simulink model "RobotSimulation"  (R2018b)
settings: Solver=VariableStepAuto  StartTime=0.0  StopTime=1  RelTol=1e-3
values from neighbouring files (symbols this model uses):
  jointAngle = inverseKinematic.ComputeInverseKinematic(jointAngle, endPose)    [CartesianTrajectoryGeneration.m]
  jointAngleStart = [175.0; 145.0; 178.0; 90.0; 180.0; 215.0; 260.0]    [CartesianTrajectoryGeneration.m]
settings Model: Creator=olavoie  LastModifiedBy=olavoie

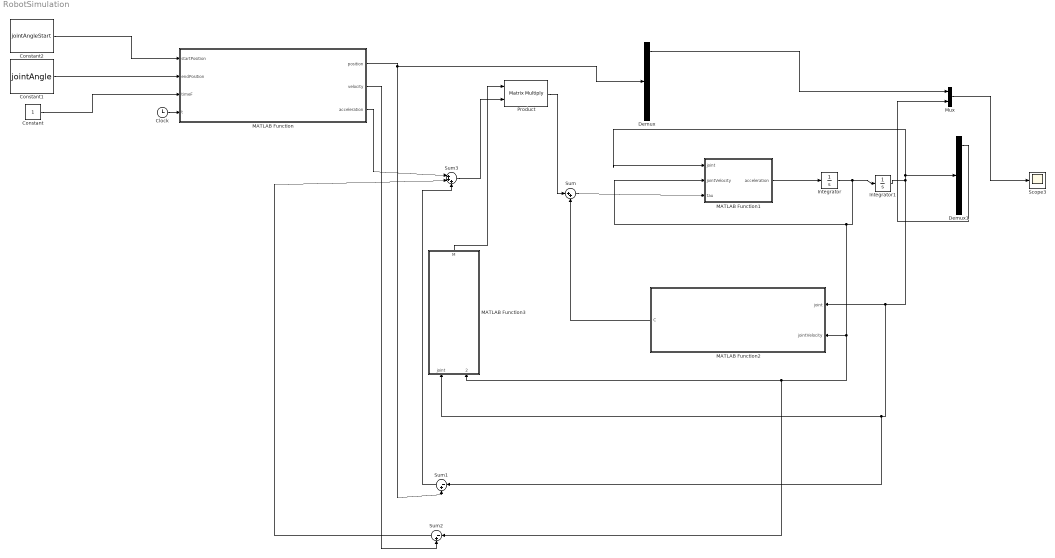
== system RobotSimulation ==
  Clock : Clock
  Constant : Constant
  Constant1 : Constant  Value=jointAngle
  Constant2 : Constant  Value=jointAngleStart
  Demux : Demux  Outputs=7
  Demux1 : Demux  Outputs=7
  Integrator : Integrator
  Integrator1 : Integrator  InitialCondition=175
  MATLAB Function : MATLAB Function  TreatAsAtomicUnit=on
  MATLAB Function1 : MATLAB Function  TreatAsAtomicUnit=on
  MATLAB Function2 : MATLAB Function  TreatAsAtomicUnit=on
  MATLAB Function3 : MATLAB Function  TreatAsAtomicUnit=on
  Mux : Mux  Inputs=2
  Product : Product  Multiplication=Matrix(*)
  Scope3 : Scope
  Sum : Sum  Inputs=|++
  Sum1 : Sum  Inputs=|-+
  Sum2 : Sum  Inputs=|-+
  Sum3 : Sum  Inputs=|+++
  wires:
  Clock/1 -> MATLAB Function/4(t)
  Constant/1 -> MATLAB Function/3(timeF)
  Constant2/1 -> MATLAB Function/1(startPosition)
  Constant1/1 -> MATLAB Function/2(endPosition)
  MATLAB Function1/1(acceleration) -> Integrator/1
  Integrator1/1 -> Demux1/1, MATLAB Function1/1(joint), Sum1/1, MATLAB Function3/1(joint), MATLAB Function2/1(joint)
  Integrator/1 -> Sum2/1, MATLAB Function3/2(jointVelocity), MATLAB Function2/2(jointVelocity), MATLAB Function1/2(jointVelocity), Integrator1/1
  MATLAB Function2/1(C) -> Sum/2
  Sum/1 -> MATLAB Function1/3(tau)
  MATLAB Function/1(position) -> Demux/1, Sum1/2
  MATLAB Function/2(velocity) -> Sum2/2
  MATLAB Function/3(acceleration) -> Sum3/1
  Sum2/1 -> Sum3/2
  Sum1/1 -> Sum3/3
  Product/1 -> Sum/1
  Sum3/1 -> Product/2
  MATLAB Function3/1(M) -> Product/1
  Mux/1 -> Scope3/1
  Demux/1 -> Mux/1
  Demux1/1 -> Mux/2

== matlab function RobotSimulation/MATLAB Function1 ==
  data: joint input; acceleration output; jointVelocity input; tau input
function acceleration = ForwardDynamicSolver(joint, jointVelocity, tau)
    % Robot Frame
    acceleration = zeros(size(tau));
    
    robotData = RobotParam;
    
    % Mass Center
    Pc = zeros(3,7);
    Pc(:, 1) = [ -3.94e-06;  0.001804699;  -0.0748562];
    Pc(:, 2) = [2.2339e-05;   0.07515658;  -0.0301928];
    Pc(:, 3) = [-2.234e-05;  0.009582299;  -0.0966774];
    Pc(:, 4) = [-3.269e-05;   0.09546485;  -0.0287837];
    Pc(:, 5) = [6.4423e-05;  -0.00987523;  -0.0607337];
    Pc(:, 6) = [5.6819e-05;   0.04279498; -0.00982194];
    Pc(:, 7) = [         0;       -2e-05;    -0.01702];

    % Mass
    m = [1.290800 1.344200 1.344200 1.094520 0.590200 0.590200 0.239480];

    % Inertia
    I = zeros(3, 3,7);
    I(:, :, 1) = [101, 0, 0; 0, 101, 0; 0, 0, 101];
    I(:, :, 2) = [102, 0, 0; 0, 102, 0; 0, 0, 102];
    I(:, :, 3) = [103, 0, 0; 0, 103, 0; 0, 0, 103];
    I(:, :, 4) = [104, 0, 0; 0, 104, 0; 0, 0, 104];
    I(:, :, 5) = [105, 0, 0; 0, 105, 0; 0, 0, 105];
    I(:, :, 6) = [106, 0, 0; 0, 106, 0; 0, 0, 106];
    I(:, :, 7) = [107, 0, 0; 0, 107, 0; 0, 0, 107];

    R = zeros(3, 3, robotData.mActuatorCount + 1);
    P = zeros(3, robotData.mActuatorCount + 1);

    % Robot referential
    for n = 1:robotData.mActuatorCount
        T = robotData.mJointReferentiel(:, :, n) * rotm2tform(rotz(joint(n) + robotData.mJointOffset(n)));
        R(:, :, n) = tform2rotm(T);
        P(:, n)    = tform2trvec(T);
    end
    
    R(:, :, robotData.mActuatorCount + 1) = [1, 0, 0; 0, 1, 0; 0, 1, 0];
    P(:, robotData.mActuatorCount + 1)    = [0; 0; 0];

    C = InverseDynamicSolver(R, P, Pc, I, m, jointVelocity, [0; 0; 0; 0; 0; 0; 0; 0], robotData.mActuatorCount)';

    M = zeros(7,7);
    for n = 1:robotData.mActuatorCount
        a = [0; 0; 0; 0; 0; 0; 0];
        a(n) = 1;
        M(:, n) = InverseDynamicSolver(R, P, Pc, I, m, jointVelocity, a, robotData.mActuatorCount)' - C;
    end 
    acceleration = inv(M) * (tau - C);
end

== matlab function RobotSimulation/MATLAB Function ==
  data: startPosition input; position output; endPosition input; timeF input; t input; velocity output; acceleration output
function  [position, velocity, acceleration] = Trajectory(startPosition, endPosition, timeF, t)

    position = zeros(size(startPosition));
    velocity = zeros(size(startPosition));
    acceleration = zeros(size(startPosition));

    for i = 1:length(startPosition)    
        S      = [startPosition(i); 0; 0; endPosition(i); 0; 0];
        M      = [1 0 0 0 0 0; 0 1 0 0 0 0; 0 0 2 0 0 0; 1 timeF timeF^2 timeF^3 timeF^4 timeF^5; 0 1 2*timeF 3*timeF^2 4*timeF^3 5*timeF^4; 0 0 2 (3*2)*timeF 4*3*timeF^2 5*4*timeF^3];

        a = M^-1 * S;
        
        position(i)     = a(1) + a(2) * t + a(3) * t^2 + a(4) * t^3 + a(5) * t^4 + a(6) * t^5;
        velocity(i)     = a(2) + 2 * a(3) * t + 3 * a(4) * t^2 + 4 * a(5) * t^3 + 5 * a(6) * t^4;
        acceleration(i) = 2 * a(3) + (3 * 2) * a(4) * t + (4 * 3) * a(5) * t^2 + (4 * 5) * a(6) * t^3;
    end

== matlab function RobotSimulation/MATLAB Function2 ==
  data: joint input; C output; jointVelocity input
function C = SystemCompensation(joint, jointVelocity)
    % Robot Frame
    acceleration = zeros(size(jointVelocity));
    
    robotData = RobotParam;
    
    % Mass Center
    Pc = zeros(3,7);
    Pc(:, 1) = [ -3.94e-06;  0.001804699;  -0.0748562];
    Pc(:, 2) = [2.2339e-05;   0.07515658;  -0.0301928];
    Pc(:, 3) = [-2.234e-05;  0.009582299;  -0.0966774];
    Pc(:, 4) = [-3.269e-05;   0.09546485;  -0.0287837];
    Pc(:, 5) = [6.4423e-05;  -0.00987523;  -0.0607337];
    Pc(:, 6) = [5.6819e-05;   0.04279498; -0.00982194];
    Pc(:, 7) = [         0;       -2e-05;    -0.01702];

    % Mass
    m = [1.290800 1.344200 1.344200 1.094520 0.590200 0.590200 0.239480];

    % Inertia
    I = zeros(3, 3,7);
    I(:, :, 1) = [101, 0, 0; 0, 101, 0; 0, 0, 101];
    I(:, :, 2) = [102, 0, 0; 0, 102, 0; 0, 0, 102];
    I(:, :, 3) = [103, 0, 0; 0, 103, 0; 0, 0, 103];
    I(:, :, 4) = [104, 0, 0; 0, 104, 0; 0, 0, 104];
    I(:, :, 5) = [105, 0, 0; 0, 105, 0; 0, 0, 105];
    I(:, :, 6) = [106, 0, 0; 0, 106, 0; 0, 0, 106];
    I(:, :, 7) = [107, 0, 0; 0, 107, 0; 0, 0, 107];

    R = zeros(3, 3, robotData.mActuatorCount + 1);
    P = zeros(3, robotData.mActuatorCount + 1);

    % Robot referential
    for n = 1:robotData.mActuatorCount
        T = robotData.mJointReferentiel(:, :, n) * rotm2tform(rotz(joint(n) + robotData.mJointOffset(n)));
        R(:, :, n) = tform2rotm(T);
        P(:, n)    = tform2trvec(T);
    end
    
    R(:, :, robotData.mActuatorCount + 1) = [1, 0, 0; 0, 1, 0; 0, 1, 0];
    P(:, robotData.mActuatorCount + 1)    = [0; 0; 0];

    C = InverseDynamicSolver(R, P, Pc, I, m, jointVelocity, [0; 0; 0; 0; 0; 0; 0; 0], robotData.mActuatorCount)';
end

== matlab function RobotSimulation/MATLAB Function3 ==
  data: joint input; M output; jointVelocity input
function M = MassMatrix(joint, jointVelocity)
    % Robot Frame    
    robotData = RobotParam;
    
    % Mass Center
    Pc = zeros(3,7);
    Pc(:, 1) = [ -3.94e-06;  0.001804699;  -0.0748562];
    Pc(:, 2) = [2.2339e-05;   0.07515658;  -0.0301928];
    Pc(:, 3) = [-2.234e-05;  0.009582299;  -0.0966774];
    Pc(:, 4) = [-3.269e-05;   0.09546485;  -0.0287837];
    Pc(:, 5) = [6.4423e-05;  -0.00987523;  -0.0607337];
    Pc(:, 6) = [5.6819e-05;   0.04279498; -0.00982194];
    Pc(:, 7) = [         0;       -2e-05;    -0.01702];

    % Mass
    m = [1.290800 1.344200 1.344200 1.094520 0.590200 0.590200 0.239480];

    % Inertia
    I = zeros(3, 3,7);
    I(:, :, 1) = [101, 0, 0; 0, 101, 0; 0, 0, 101];
    I(:, :, 2) = [102, 0, 0; 0, 102, 0; 0, 0, 102];
    I(:, :, 3) = [103, 0, 0; 0, 103, 0; 0, 0, 103];
    I(:, :, 4) = [104, 0, 0; 0, 104, 0; 0, 0, 104];
    I(:, :, 5) = [105, 0, 0; 0, 105, 0; 0, 0, 105];
    I(:, :, 6) = [106, 0, 0; 0, 106, 0; 0, 0, 106];
    I(:, :, 7) = [107, 0, 0; 0, 107, 0; 0, 0, 107];

    R = zeros(3, 3, robotData.mActuatorCount + 1);
    P = zeros(3, robotData.mActuatorCount + 1);

    % Robot referential
    for n = 1:robotData.mActuatorCount
        T = robotData.mJointReferentiel(:, :, n) * rotm2tform(rotz(joint(n) + robotData.mJointOffset(n)));
        R(:, :, n) = tform2rotm(T);
        P(:, n)    = tform2trvec(T);
    end
    
    R(:, :, robotData.mActuatorCount + 1) = [1, 0, 0; 0, 1, 0; 0, 1, 0];
    P(:, robotData.mActuatorCount + 1)    = [0; 0; 0];

    C = InverseDynamicSolver(R, P, Pc, I, m, jointVelocity, [0; 0; 0; 0; 0; 0; 0; 0], robotData.mActuatorCount)';

    M = zeros(7,7);
    for n = 1:robotData.mActuatorCount
        a = [0; 0; 0; 0; 0; 0; 0];
        a(n) = 1;
        M(:, n) = InverseDynamicSolver(R, P, Pc, I, m, jointVelocity, a, robotData.mActuatorCount)' - C;
    end 
end
